simulink model "single_MSM_tooth_simulation"  (R2022b)
settings: Solver=ode23  StartTime=0.0  StopTime=SIMULATION_TIME  FixedStep=MAX_TIME_STEP  MaxStep=MAX_TIME_STEP  RelTol=1e-3  AbsTol=1e-3  EnableMultiTasking=on
values from neighbouring files (symbols this model uses):
  contraction_initial = -msm_length * e_initial    (= -0.0005)    [MSM_mechanism_simulation_properties.m]
  min_tooth_motion_range = -msm_length * allowed_elongation    (= -0.0005)    [MSM_mechanism_simulation_properties.m]
  one_side_absolute_offset = one_side_elongation_capacity * msm_length    (= 5e-05)    [MSM_mechanism_simulation_properties.m]
  rand_seed_1 = randi([1 1e+7])    [msm_tooth_training_run.m]
  rand_seed_2 = randi([1 1e+7])    [msm_tooth_training_run.m]
  sine_phase = randi([1 1e+10]) / 100    [msm_tooth_training_run.m]
  tooth_random_initial_pos_coefficient = get_rand_initial_position()    [msm_tooth_training_run.m]
  trajectory_mode = randi([0 2])    [msm_tooth_training_run.m]
  Z = griddata(x,y,z,X,Y)    [MSM_simulation_data_processing.m]
undefined symbols (not defined in the file or in its folder): control_input, sigbuilder_block, X, Y
libraries: sm_lib x5, deeplib x3, simulink x2, nesl_utility x2, Flat_tooth_plate x1, MSM_element x1
settings Model: Creator=h19343  LastModifiedBy=h19343
settings SolverCC: AutoScaleAbsTol=off  MaxZcPerStep=1
settings DataIOCC: LimitDataPoints=on  MaxDataPoints=10000
settings OptimizationCC: LifeSpan=inf
settings DebuggingCC: AlgebraicLoopMsg=none  UnconnectedInputMsg=warning  AllowSymbolicDim=off  SFUnexpectedBacktrackingDiag=warning  SFNoUnconditionalDefaultTransitionDiag=warning  SFExecutionAtInitializationDiag=none  SFMachineParentedDataDiag=warning  ArithmeticOperatorsInVariantConditions=warning
settings ModelReferenceCC: EnableRefExpFcnMdlSchedulingChecks=on
settings SFSimCC: SimUseLocalCustomCode=off  CustomCodeUndefinedFunction=UseInterfaceOnly
settings RTWCC: RTWUseLocalCustomCode=off  DLArmComputeVersion=19.05
settings CodeAppCC: StateflowObjectComments=on
settings GRTTargetCC: TargetLangStandard=C89/C90 (ANSI)
settings ConfigComp: CovMetricSettings=dw  CovSaveCumulativeToWorkspaceVar=on  CovSaveSingleToWorkspaceVar=on  CovExternalEMLEnable=off  CovSFcnEnable=off
settings SimscapeCC: ExplicitSolverDiagnosticOptions=none  SimscapeLogType=all  SimscapeLogSimulationStatistics=on  SimscapeLogDataHistory=10000

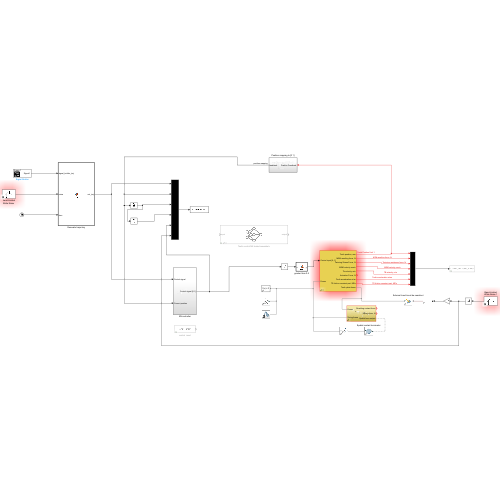
[thumbnail: Simulink's stored preview of the top-level diagram]
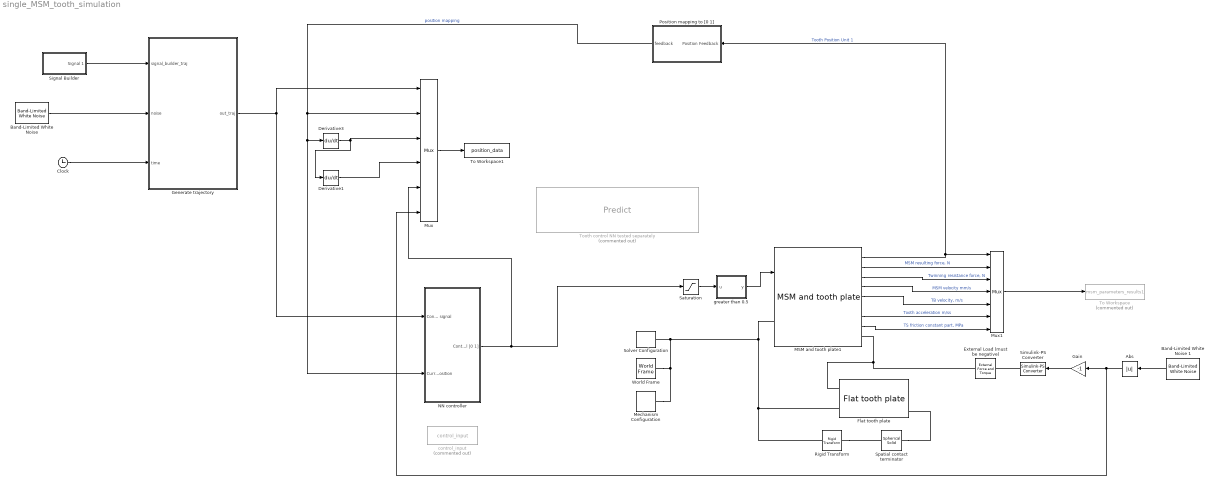
== system single_MSM_tooth_simulation ==
  Abs : Abs  SaturateOnIntegerOverflow=off
  "Band-Limited White Noise " : simulink/Sources/Band-Limited White Noise  Cov=[1e-9]  Ts=5e-4  seed=[rand_seed_1]
  Band-Limited White Noise 1 : simulink/Sources/Band-Limited White Noise  Cov=[1e-3]  Ts=1e-3  seed=[rand_seed_2]
  Clock : Clock
  Derivative1 : Derivative
  Derivative3 : Derivative
  External Load (must be negative) : sm_lib/Forces and Torques/External Force and Torque  ForceResolutionFrame=AttachedFrame  EnableForceX=off  EnableForceY=on  EnableForceZ=off  EnableForce=off  TorqueResolutionFrame=AttachedFrame  EnableTorqueX=off  EnableTorqueY=off  EnableTorqueZ=off  EnableTorque=off
  Flat tooth plate : Flat_tooth_plate/Flat tooth plate  SystemSampleTime=-1  VariantActivationTime=update diagram  Latency=0  AutoFrameSizeCalculation=off
  Gain : Gain  Gain=-1
  Generate trajectory : MATLAB Function  TreatAsAtomicUnit=on
  MSM and tooth plate1 : MSM_element/MSM and tooth plate  PositionTargetValue=contraction_initial * tooth_random_initial_pos_coefficient
  Mechanism Configuration : sm_lib/Utilities/Mechanism Configuration  UniformGravity=Constant  GravityVector=[0 0 0]  GravityUnits=m/s^2  LinearizationDelta=0.001  JointModeTransitionNonlinearIterations=2
  Mux : Mux  Inputs=6
  Mux1 : Mux  Inputs=7
  NN controller : Subsystem
  Position mapping to [0 1] : Subsystem
  Rigid Transform : sm_lib/Frames and Transforms/Rigid Transform  TranslationMethod=Cartesian  TranslationStandardOffset=0  TranslationLengthUnit=m  TranslationStandardAxis=+Z  TranslationCartesianOffset=[0 -0.01 0]  TranslationROffset=0  TranslationROffsetUnits=m  TranslationZOffset=0  TranslationZOffsetUnits=m  TranslationThetaOffset=0  TranslationThetaOffsetUnits=deg  RotationMethod=None  RotationAngleUnits=deg  RotationStandardAxis=+Z  RotationAngle=0.0  RotationArbitraryAxis=[0 0 1]  FollAlignAxisA=+X  BaseAlignAxisA=+Y  FollAlignAxisB=+Y  BaseAlignAxisB=+Z  RotationSequenceAxes=FollowerAxes  RotationSequence=XYX  RotationSequenceAngles=[0 0 0]  RotationSequenceAnglesUnits=deg  RotationMatrix=[1 0 0; 0 1 0; 0 0 1]  Quaternion=[1 0 0 0]
  Saturation : Saturate  UpperLimit=1  LowerLimit=0
  Signal Builder : Subsystem  Tag=STV Subsys  LoadFcn=sigbuilder_block('load');  StartFcn=sigbuilder_block('start');  StopFcn=sigbuilder_block('stop');  ClipboardFcn=sigbuilder_block('clipboard');  mask(Sigbuilder block){tuvar=[0:10]}
      mask help: Simulink:masks:SigbuilderBlock_MD
      mask init:
      | if ~strcmp(get_param(bdroot(gcbh),'SimulationStatus'),'stopped') tuvar = sigbuilder_block('maskInit'); end
      settings: CopyFcn=sigbuilder_block('copy');  DeleteFcn=sigbuilder_block('delete');  ModelCloseFcn=sigbuilder_block('modelClose');  PreSaveFcn=sigbuilder_block('preSave');  PauseFcn=sigbuilder_block('pause');  ContinueFcn=sigbuilder_block('continue');  NameChangeFcn=sigbuilder_block('namechange');  OpenFcn=sigbuilder_block('open',[121.2 94.2 550.8 400.2 ]);  CloseFcn=sigbuilder_block('close');
      mask Display: plot(0, 0, 100, 100,[2, 2, 32, 32, 2], [68, 8, 8, 68, 68],[32, 2], [38, 38], [32, 19, 2],[53, 60, 44], [32, 17, 17, 2],[16, 16, 31, 31]);txt = getActiveGroup(gcbh);text(2, 100, txt,'verticalAlignment', 'top');
  Simulink-PS Converter : nesl_utility/Simulink-PS Converter  PhysicalDomain=network_engine_domain  SubClassName=ps_input  LeftPortType=input  RightPortType=output  PseudoPeriodic=off  Frequencies=[]  NoiseDistribution=none  NoiseParameters=[]  Unit=N  AffineConversion=off  FilteringAndDerivatives=provide  SimscapeFilterOrder=2  InputFilterTimeConstant=0.001  UdotUserProvided=0
  Solver Configuration : nesl_utility/Solver Configuration  PhysicalDomain=network_engine_domain  SubClassName=solver  LeftPortType=input  RightPortType=generic  Tones=[]  Harmonics=[]  SimulateNoise=off  Profile=off  UseLocalSampling=off  EnableSwitchedLinearOptims=on  FrequencyDomain=off  UseCCode=off  RelTol=0.001  AbsTol=1e-06  MinStep=1e-09  ToWorkspace=off  RevertToSquareIcSolve=off  NumHomotopyIterations=100  PhasorMode=off  PhasorModeNumHarmonics=1  ConsistencySolver=NEWTON_FTOL  IndexReductionMethod=DerivativeReplacement  DoDC=off  ResidualTolerance=1e-09  ConsistencyTolSource=GLOBAL  ConsistencyAbsTol=0.001  ConsistencyRelTol=0.001  ConsistencyTolFactor=0.001  UseLocalSolver=off  LocalSolverChoice=NE_BACKWARD_EULER_ADVANCER  ResolveIndetEquations=on  FunctionEvalNumThread=1  LocalSolverSampleTime=0.001  DoFixedCost=off  MaxNonlinIter=3  MaxModeIter=2  ComputeImpulses=off  ImpulseIterations=2  LinearAlgebra=Sparse  LinearAlgebraNumThread=0  EquationFormulation=NE_TIME_EF  DelaysMemoryBudget=1024  AutomaticFiltering=on  FilteringTimeConstant=0.001  PartitionStorageMethod=AS_NEEDED  PartitionMemoryBudget=1024  PartitionMethod=FAST
  Spatial contact terminator : sm_lib/Body Elements/Spherical Solid  GraphicAmbientColor=[0.15 0.15 0.15 1.0]  BasedOnType=Density  CenterOfMass=[0 0 0]  CenterOfMassUnits=m  GraphicDiffuseColor=[1.0 0.2 0.2]  Density=1000  DensityUnits=kg/m^3  DoExposeReferenceFrame=on  GraphicEmissiveColor=[0.0 0.0 0.0 1.0]  ExportEntireGeometry=on  SerializedExposedGeometries=<ExposedGeometries><ExposedGeometry><RawGeometryId>entire</RawGeometryId><ExposedGeometryId>G</ExposedGeometryId></ExposedGeometry></ExposedGeometries>  SerializedFrames=<Frames/>  MarkerShape=Sphere  MarkerSize=10  GraphicType=FromGeometry  InertiaType=CalculateFromGeometry  Mass=1  MassUnits=kg  MomentsOfInertia=[1 1 1]  MomentsOfInertiaUnits=kg*m^2  GraphicOpacity=1.0  ProductsOfInertia=[0 0 0]  ProductsOfInertiaUnits=kg*m^2  GraphicShininess=75  GraphicSpecularColor=[0.5 0.5 0.5 1.0]  SphereRadius=0.00001  SphereRadiusUnits=m  GraphicVisPropType=SimpleVisualProperties
  To Workspace : ToWorkspace  Commented=on  VariableName=msm_parameters_results1  SaveFormat=Timeseries  SampleTime=-1
  To Workspace1 : ToWorkspace  VariableName=position_data  SaveFormat=Timeseries  SampleTime=-1
  Tooth control NN tested separately : deeplib/Predict  Commented=on  Network=Network from MAT-file  NetworkFunction=squeezenet  NetworkFilePath=net.mat  MiniBatchSize=128  InputDataFormats={'',''}  Predictions=on  Activations={}  ForceInterpretedSim=off  EnableDLNetwork=on
  World Frame : sm_lib/Frames and Transforms/World Frame
  control_input : Constant  Commented=on  Value=control_input
  greater than 0.5 : MATLAB Function  TreatAsAtomicUnit=on
  wires:
  MSM and tooth plate1/8 -> Mux1/7  "TS friction constant part, MPa"
  MSM and tooth plate1/2 -> Mux1/2  "MSM resulting force, N"
  MSM and tooth plate1/5 -> Mux1/5  "TB velocity, m/s"
  MSM and tooth plate1/3 -> Mux1/3  "Twinning resistance force, N"
  Mux1/1 -> To Workspace/1
  MSM and tooth plate1/1 -> Position mapping to [0 1]/1(Position Feedback), Mux1/1  "Tooth Position Unit 1"
  MSM and tooth plate1/4 -> Mux1/4  "MSM velocity mm/s"
  MSM and tooth plate1/7 -> Mux1/6  "Tooth acceleration m/ss"
  Position mapping to [0 1]/1(feedback) -> NN controller/2(Current position), Derivative3/1, Mux/2  "position mapping"
  Saturation/1 -> greater than 0.5/1(u)
  Mux/1 -> To Workspace1/1
  Generate trajectory/1(out_traj) -> Mux/1, NN controller/1(Control signal)
  greater than 0.5/1(y) -> MSM and tooth plate1/1
  Derivative3/1 -> Derivative1/1, Mux/3
  Derivative1/1 -> Mux/4
  NN controller/1(Control signal [0 1]) -> Mux/5, Saturation/1
  Abs/1 -> Mux/6, Gain/1
  Gain/1 -> Simulink-PS Converter/1
  Band-Limited White Noise 1/1 -> Abs/1
  Signal Builder/1(Signal 1) -> Generate trajectory/1(signal_builder_traj)
  "Band-Limited White Noise "/1 -> Generate trajectory/2(noise)
  Clock/1 -> Generate trajectory/3(time)
  connections:
  MSM and tooth plate1/LConn1 -- Rigid Transform/LConn1 -- Flat tooth plate/LConn2 -- Mechanism Configuration/RConn1 -- World Frame/RConn1 -- Solver Configuration/RConn1
  Flat tooth plate/LConn1 -- MSM and tooth plate1/RConn1 -- External Load (must be negative)/RConn1
  Spatial contact terminator/LConn1 -- Flat tooth plate/RConn1
  Rigid Transform/RConn1 -- Spatial contact terminator/RConn1
  Simulink-PS Converter/RConn1 -- External Load (must be negative)/LConn1

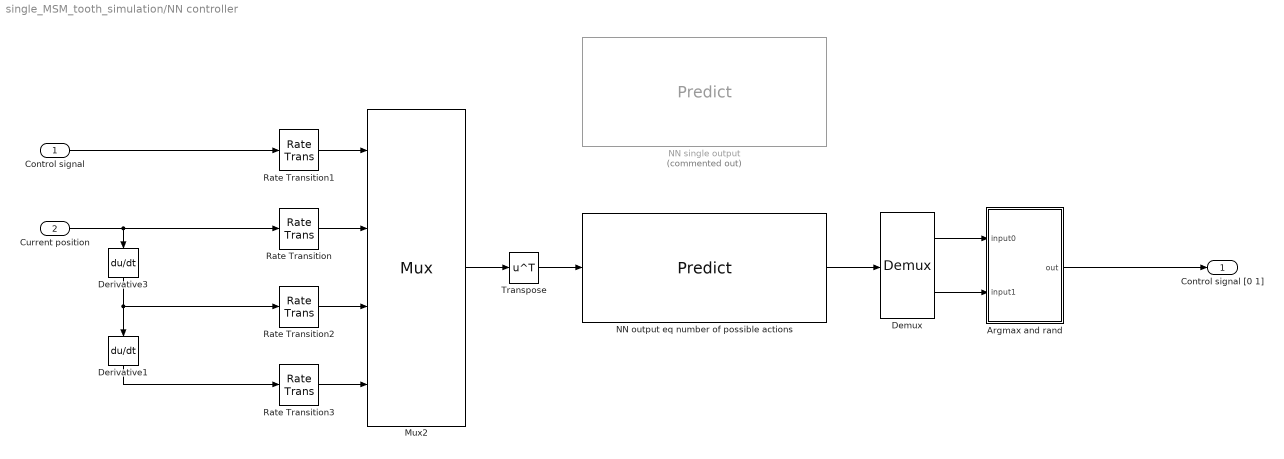
== system single_MSM_tooth_simulation/NN controller ==
  Control signal : Inport
  Current position : Inport  Port=2
  Argmax and rand : MATLAB Function  TreatAsAtomicUnit=on
  Demux : Demux  Outputs=2
      settings: DisplayOption=none
  Derivative1 : Derivative
  Derivative3 : Derivative
  Mux2 : Mux
      settings: DisplayOption=signals
  NN output eq number of possible actions : deeplib/Predict  Network=Network from MAT-file  NetworkFunction=squeezenet  NetworkFilePath=net.mat  MiniBatchSize=1  InputDataFormats={'',''}  Predictions=on  Activations={}  ForceInterpretedSim=off  EnableDLNetwork=on
  NN single output : deeplib/Predict  Commented=on  Network=Network from MAT-file  NetworkFunction=squeezenet  NetworkFilePath=net.mat  MiniBatchSize=1  InputDataFormats={'',''}  Predictions=on  Activations={}  ForceInterpretedSim=off  EnableDLNetwork=on
  Rate Transition{,1..3} (4 alike) : RateTransition  OutPortSampleTime=1e-6
  Transpose : Math  Operator=transpose
  Control signal [0 1] : Outport
  wires:
  Rate Transition2/1 -> Mux2/3
  Rate Transition3/1 -> Mux2/4
  Derivative3/1 -> Derivative1/1, Rate Transition2/1
  Rate Transition/1 -> Mux2/2
  Transpose/1 -> NN output eq number of possible actions/1
  Rate Transition1/1 -> Mux2/1
  Mux2/1 -> Transpose/1
  Control signal/1 -> Rate Transition1/1
  Current position/1 -> Derivative3/1, Rate Transition/1
  Derivative1/1 -> Rate Transition3/1
  NN output eq number of possible actions/1 -> Demux/1
  Demux/1 -> Argmax and rand/1(input0)
  Demux/2 -> Argmax and rand/2(input1)
  Argmax and rand/1(out) -> Control signal [0 1]/1

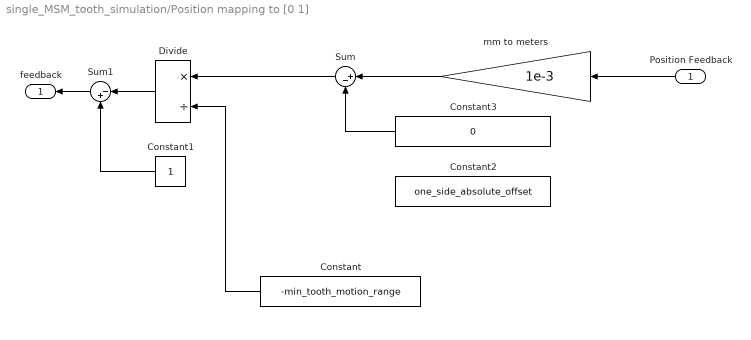
== system single_MSM_tooth_simulation/Position mapping to [0 1] ==
  Position Feedback : Inport
  Constant : Constant  Value=-min_tooth_motion_range
  Constant1 : Constant
  Constant2 : Constant  Value=one_side_absolute_offset
  Constant3 : Constant  Value=0
  Divide : Product  Inputs=*/
  Sum : Sum  Inputs=|+-
  Sum1 : Sum  Inputs=|-+
  mm to meters : Gain  Gain=1e-3
  feedback : Outport
  wires:
  Position Feedback/1 -> mm to meters/1
  Sum/1 -> Divide/1
  Constant/1 -> Divide/2
  Divide/1 -> Sum1/1
  Sum1/1 -> feedback/1
  Constant1/1 -> Sum1/2
  mm to meters/1 -> Sum/1
  Constant3/1 -> Sum/2

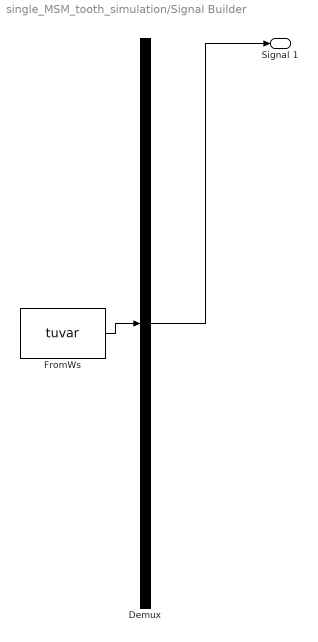
== system single_MSM_tooth_simulation/Signal Builder ==
  Demux : Demux  Tag=STV Demux  Outputs=1
      settings: DisplayOption=none
  FromWs : FromWorkspace  Tag=STV FromWs  VariableName=tuvar
      SigBuilderData=|
      | common.afterFinalStr = 'Extrapolate'
      | common.sampleTime = 0
      | dataSet.timeRange = [0 0.06]
      | dataSet.name = 'Group 1'
      | sbobj.Groups.Name = 'Group 1'
      | sbobj.Groups.Signals.Name = 'Signal 1'
      | sbobj.Groups.Signals.XData = [0 0.007 0.0086 0.0098 0.011 0.0118 0.0166 0.0182 0.021 0.024 0.026 0.028 0.0304 0.0322 0.0344 0.0362 0.0378 0.04 0.0438 0.045 0.0472 0.0492 0.0532 0.0547 0.0559 0.0572 0.06]
      | sbobj.Groups.Signals.YData = [0.045 0.97 0.97 0.895 0.81 0.85 0.42 0.42 0.03 0.18 0.105 0.19 0.135 0.26 0.235 0.315 0.295 0.39 0.59 0.98 0.98 0.045 0.045 0.209338235294 0.315 0.185 0.58]
      | sbobj.Groups.TimeRange = [0 0.06]
  Signal 1 : Outport  Tag=STV Outport
  wires:
  Demux/1 -> Signal 1/1
  FromWs/1 -> Demux/1

== matlab function single_MSM_tooth_simulation/greater than 0.5 ==
  data: u input; y output
function y = fcn(u)
if u > 0.5
    y = 1;
else
    y = 0;
end

== matlab function single_MSM_tooth_simulation/NN controller/Argmax and rand ==
  data: input0 input; out output; input1 input; epsilon parameter
function out = fcn(input0, input1, epsilon)

if rand < epsilon
    out = round(rand);
    return;
end

if input0 > input1
    out = 0;
else
    out = 1;
end

end

== matlab function single_MSM_tooth_simulation/Generate trajectory ==
  data: signal_builder_traj input; out_traj output; noise input; time input; sine_phase parameter; trajectory_mode parameter
function out_traj = fcn(signal_builder_traj, noise, time, sine_phase, trajectory_mode)

if trajectory_mode < 0.5
    out_traj = signal_builder_traj + noise;
elseif trajectory_mode < 1.5
    out_traj = 0.5 + 0.45 * sin(150*time + sine_phase);
else
    out_traj = 0.5 + noise * 80;
end

out_traj = max(0.02, out_traj);
out_traj = min(0.98, out_traj);

end
